simulink model "sampleModel3"  (R2023a)
settings: Solver=FixedStepAuto  StartTime=0.0  StopTime=10.0  RelTol=1e-3
undefined symbols (not defined in the file): DiscIntNeverNeededParam
libraries: simulink x8
settings Model: SimulationMode=software-in-the-loop (sil)  Creator=TSMC  LastModifiedBy=O
settings DataIOCC: InspectSignalLogs=on  SignalLoggingName=logsOut
settings OptimizationCC: DefaultParameterBehavior=Inlined  EnhancedBackFolding=on  PassReuseOutputArgsAs=Individual arguments  ZeroExternalMemoryAtStartup=off  ZeroInternalMemoryAtStartup=off  OptimizeBlockOrder=speed  DifferentSizesBufferReuse=on  OptimizationCustomize=off  EfficientTunableParamExpr=on
settings DebuggingCC: ParameterTunabilityLossMsg=error
settings ModelReferenceCC: UpdateModelReferenceTargets=Force
settings SFSimCC: MATLABDynamicMemAlloc=off
settings RTWCC: Description=Embedded Coder  SystemTargetFile=ert.tlc  TemplateMakefile=ert_default_tmf  GenerateReport=on  IncludeHyperlinkInReport=on  GenerateTraceInfo=on
settings CodeAppCC: ForceParamTrailComments=on  IgnoreCustomStorageClasses=off  OperatorAnnotations=on  SimulinkDataObjDesc=on  SFDataObjDesc=on  InsertBlockDesc=on
settings ERTTargetCC: TargetLangStandard=C99 (ISO)  GenerateSampleERTMain=on  SupportContinuousTime=on  InlinedParameterPlacement=NonHierarchical  ERTCustomFileTemplate=example_file_process.tlc

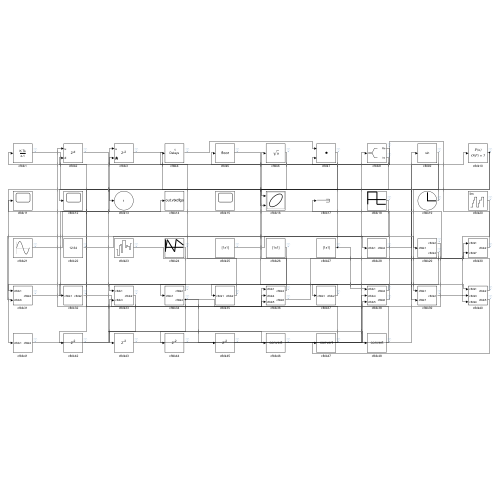
[thumbnail: Simulink's stored preview of the top-level diagram]
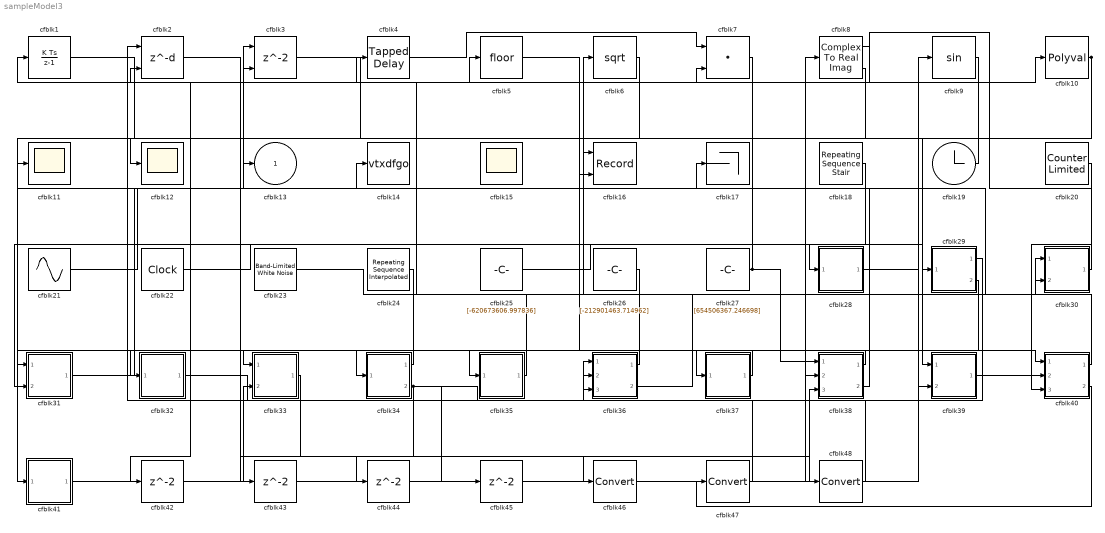
== system sampleModel3 ==
  cfblk1 : DiscreteIntegrator  ICPrevOutput=DiscIntNeverNeededParam  ICPrevScaledInput=DiscIntNeverNeededParam
  cfblk10 : Polyval  Coefs=[ +2.081618890e-019, -1.441693666e-014, +4.719686976e-010, -8.536869453e-006, +1.621573104e-001, -8.087801117e+001 ]
  cfblk11 : Scope
  cfblk12 : Scope
  cfblk14 : ToWorkspace  VariableName=vtxdfgo  SaveFormat=Timeseries  SampleTime=-1
  cfblk15 : Scope
      settings: Floating=on
  cfblk16 : Record  FileSettingsInternal="{\"entries\":[{\"content\":{\"excelSettings\":{\"content\":{},\"type\":\"Streamout.ExcelSettings\"}},\"type\":\"Streamout.FileSettingStorage\",\"uuid\":\"\"}],\"packageUris\":[\"http:\\/\\/schema.mathworks.com\\/mf0\\/streamout_blocks\\/R2020a\"],\"version\":\"1.0\"}"  Layout=[1 1]  SignalsInternal="{\"entries\":[{\"content\":{},\"type\":\"RecordBlkView.InputSignals\",\"uuid\":\"\"}],\"packageUris\":[\"http:\\/\\/schema.mathworks.com\\/mf0\\/streamout_blocks\\/R2020a\"],\"version\":\"1.0\"}"  VisualizationBindings="{\"xyplotplugin\":{\"info\":[{\"series\":[],\"subplotID\":1}]}}"  CompatibilityTag=XY
  cfblk17 : Terminator
  cfblk18 : simulink/Sources/Repeating Sequence Stair  OutValues=[683621746.226456, -425976951.351904]  tsamp=-1  OutMin=[]  OutMax=[]  OutDataTypeStr=double  OutputDataTypeScalingMode=double  OutDataType=fixdt(0,8)  ConRadixGroup=Best Precision: Vector-wise  OutScaling=2^-12
  cfblk19 : Clock
  cfblk2 : Delay  DelayLengthSource=Input port  SampleTime=1
      settings: InputPortMap=u0,p1
  cfblk20 : simulink/Sources/Counter Limited  uplimit=[952.000000]  tsamp=-1
  cfblk21 : Sin  Amplitude=[-7935361.579874]  Bias=[-620617910.021881]  SampleTime=0
  cfblk22 : DigitalClock
  cfblk23 : simulink/Sources/Band-Limited White Noise  Cov=[6099696625.296525]  Ts=0.1  seed=[892437433.000000]
  cfblk24 : simulink/Sources/Repeating Sequence Interpolated  OutValues=[-241246574.591498, 696589319.816223, -385466579.888859, 738540772.588338, 209128853.728495]  TimeValues=[0 0.1 0.5 0.6 1].'  LookUpMeth=Use Input Nearest  tsamp=0.01  OutMin=[]  OutMax=[]  OutDataTypeStr=double  OutputDataTypeScalingMode=double  OutDataType=fixdt(0,8)  OutScaling=2^-10
  cfblk25 : Constant  Value=[-620673606.997836]  SampleTime=1
  cfblk26 : Constant  Value=[-212901463.714962]  SampleTime=1
  cfblk27 : Constant  Value=[654506367.246698]  SampleTime=1
  cfblk28 : Subsystem
  cfblk29 : Subsystem
  cfblk3 : Delay  ShowEnablePort=on  SampleTime=1
      settings: InputPortMap=u0,e6
  cfblk30 : Subsystem
  cfblk31 : Subsystem
  cfblk32 : Subsystem
  cfblk33 : Subsystem
  cfblk34 : Subsystem
  cfblk35 : Subsystem
  cfblk36 : Subsystem
  cfblk37 : Subsystem
  cfblk38 : Subsystem
  cfblk39 : Subsystem
  cfblk4 : simulink/Discrete/Tapped Delay  vinit=0.0  samptime=-1  NumDelays=1  DelayOrder=Oldest  includeCurrent=off
  cfblk40 : Subsystem
  cfblk41 : Subsystem
  cfblk{42..45} (4 alike) : Delay  SampleTime=1
  cfblk46 : DataTypeConversion  SaturateOnIntegerOverflow=off  RndMeth=Floor
  cfblk47 : DataTypeConversion  SaturateOnIntegerOverflow=off  RndMeth=Floor
  cfblk48 : DataTypeConversion  SaturateOnIntegerOverflow=off  RndMeth=Floor
  cfblk5 : Rounding
  cfblk6 : Sqrt
  cfblk7 : DotProduct  OutDataTypeStr=Inherit: Inherit via internal rule
  cfblk8 : ComplexToRealImag
  cfblk9 : Trigonometry
  cfblk13 : Outport
  wires:
  cfblk31/1(cfblk2) -> cfblk14/1
  cfblk26/1 -> cfblk33/1(cfblk1)
  cfblk25/1 -> cfblk39/1(cfblk1)
  cfblk9/1 -> cfblk41/1(cfblk1)
  cfblk29/1(cfblk2) -> cfblk36/1(cfblk1)
  cfblk40/1(cfblk2) -> cfblk17/1
  cfblk22/1 -> cfblk28/1(cfblk1)
  cfblk29/2(cfblk4) -> cfblk35/1(cfblk1)
  cfblk3/1 -> cfblk39/2(cfblk7)
  cfblk30/1(cfblk2) -> cfblk5/1
  cfblk19/1 -> cfblk1/1
  cfblk35/1(cfblk2) -> cfblk4/1
  cfblk36/1(cfblk2) -> cfblk6/1
  cfblk21/1 -> cfblk3/1
  cfblk38/1(cfblk2) -> cfblk37/1(cfblk1)
  cfblk5/1 -> cfblk40/1(cfblk1)
  cfblk27/1 -> cfblk3/2, cfblk38/1(cfblk1)
  cfblk36/2(cfblk6) -> cfblk30/1(cfblk1)
  cfblk32/1(cfblk2) -> cfblk36/2(cfblk4)
  cfblk23/1 -> cfblk30/2(cfblk7)
  cfblk24/1 -> cfblk31/1(cfblk1)
  cfblk10/1 -> cfblk29/1(cfblk1), cfblk16/2
  cfblk4/1 -> cfblk7/1
  cfblk20/1 -> cfblk40/2(cfblk3)
  cfblk38/2(cfblk6) -> cfblk11/1
  cfblk41/1(cfblk2) -> cfblk33/2(cfblk3)
  cfblk1/1 -> cfblk13/1
  cfblk18/1 -> cfblk31/2(cfblk6)
  cfblk39/1(cfblk2) -> cfblk40/3(cfblk4)
  cfblk8/1 -> cfblk7/2
  cfblk7/1 -> cfblk16/1
  cfblk6/1 -> cfblk12/1
  cfblk28/1(cfblk2) -> cfblk10/1
  cfblk37/1(cfblk2) -> cfblk34/1(cfblk1)
  cfblk34/1(cfblk2) -> cfblk32/1(cfblk1)
  cfblk34/2(cfblk4) -> cfblk36/3(cfblk5), cfblk44/1, cfblk45/1
  cfblk8/2 -> cfblk42/1
  cfblk33/1(cfblk2) -> cfblk43/1
  cfblk43/1 -> cfblk9/1
  cfblk44/1 -> cfblk38/2(cfblk4)
  cfblk45/1 -> cfblk38/3(cfblk5)
  cfblk2/1 -> cfblk46/1
  cfblk46/1 -> cfblk8/1
  cfblk40/2(cfblk5) -> cfblk47/1
  cfblk47/1 -> cfblk2/1
  cfblk42/1 -> cfblk48/1
  cfblk48/1 -> cfblk2/2

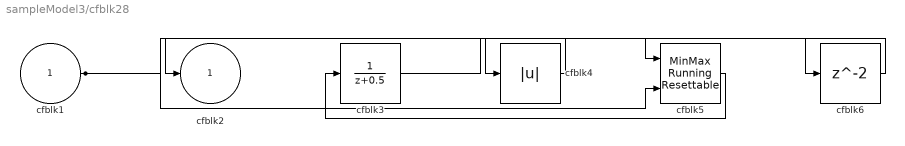
== system sampleModel3/cfblk28 ==
  cfblk1 : Inport
  cfblk3 : DiscreteTransferFcn  SampleTime=1
  cfblk4 : Abs  SaturateOnIntegerOverflow=off
  cfblk5 : simulink/Math Operations/MinMax Running Resettable  Function=min  vinit=0.0
  cfblk6 : Delay  SampleTime=1
  cfblk2 : Outport
  wires:
  cfblk4/1 -> cfblk2/1
  cfblk5/1 -> cfblk3/1
  cfblk1/1 -> cfblk5/2, cfblk4/1
  cfblk3/1 -> cfblk6/1
  cfblk6/1 -> cfblk5/1

== system sampleModel3/cfblk29 ==
  cfblk1 : Inport
  cfblk3 : Sum  Inputs=|++
  cfblk2 : Outport
  cfblk4 : Outport  Port=2
  wires:
  cfblk3/1 -> cfblk2/1
  cfblk1/1 -> cfblk4/1, cfblk3/1, cfblk3/2

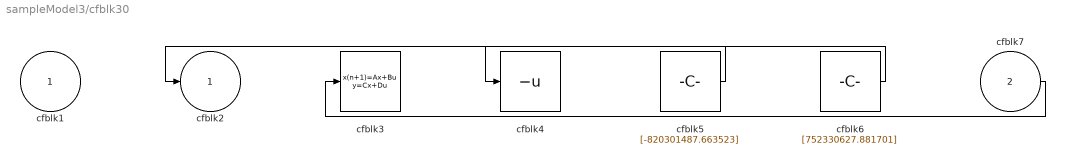
== system sampleModel3/cfblk30 ==
  cfblk1 : Inport
  cfblk7 : Inport  Port=2
  cfblk3 : DiscreteStateSpace
  cfblk4 : UnaryMinus
  cfblk5 : Constant  Value=[-820301487.663523]  SampleTime=1
  cfblk6 : Constant  Value=[752330627.881701]  SampleTime=1
  cfblk2 : Outport
  wires:
  cfblk6/1 -> cfblk4/1
  cfblk7/1 -> cfblk3/1
  cfblk5/1 -> cfblk2/1

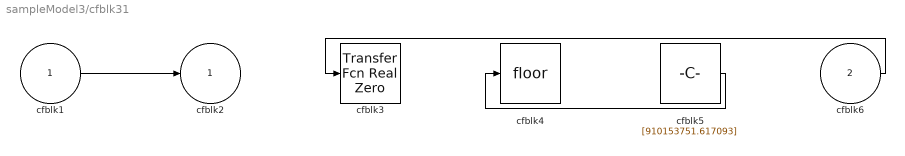
== system sampleModel3/cfblk31 ==
  cfblk1 : Inport
  cfblk6 : Inport  Port=2
  cfblk3 : simulink/Discrete/Transfer Fcn Real Zero  ZeroZ=0.75  ICPrevInput=0.0  DoSatur=off
  cfblk4 : Rounding
  cfblk5 : Constant  Value=[910153751.617093]  SampleTime=1
  cfblk2 : Outport
  wires:
  cfblk6/1 -> cfblk3/1
  cfblk5/1 -> cfblk4/1
  cfblk1/1 -> cfblk2/1

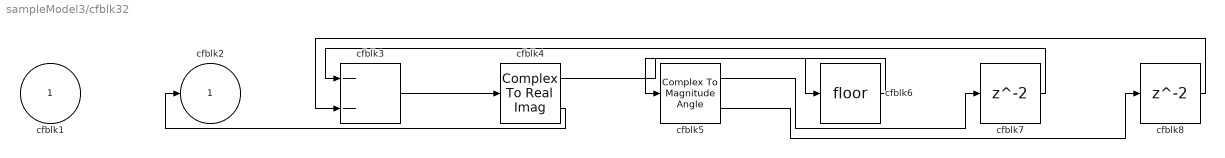
== system sampleModel3/cfblk32 ==
  cfblk1 : Inport
  cfblk3 : Sum  Inputs=--
  cfblk4 : ComplexToRealImag
  cfblk5 : ComplexToMagnitudeAngle
  cfblk6 : Rounding
  cfblk7 : Delay  SampleTime=1
  cfblk8 : Delay  SampleTime=1
  cfblk2 : Outport
  wires:
  cfblk6/1 -> cfblk5/1
  cfblk3/1 -> cfblk4/1
  cfblk4/1 -> cfblk6/1
  cfblk4/2 -> cfblk2/1
  cfblk5/1 -> cfblk7/1
  cfblk7/1 -> cfblk3/1
  cfblk5/2 -> cfblk8/1
  cfblk8/1 -> cfblk3/2

== system sampleModel3/cfblk33 ==
  cfblk1 : Inport
  cfblk3 : Inport  Port=2
  cfblk2 : Outport
  wires:
  cfblk1/1 -> cfblk2/1

== system sampleModel3/cfblk34 ==
  cfblk1 : Inport
  cfblk3 : Sum  Inputs=|++
  cfblk2 : Outport
  cfblk4 : Outport  Port=2
  wires:
  cfblk1/1 -> cfblk3/1, cfblk4/1, cfblk3/2
  cfblk3/1 -> cfblk2/1

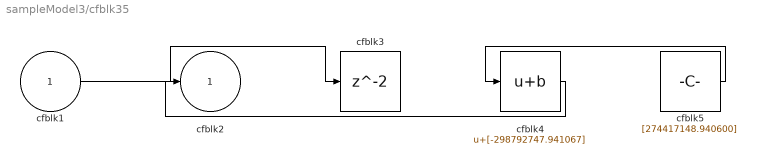
== system sampleModel3/cfblk35 ==
  cfblk1 : Inport
  cfblk3 : Delay  SampleTime=1
  cfblk4 : Bias  Bias=[-298792747.941067]  SaturateOnIntegerOverflow=off
  cfblk5 : Constant  Value=[274417148.940600]  SampleTime=1
  cfblk2 : Outport
  wires:
  cfblk5/1 -> cfblk4/1
  cfblk1/1 -> cfblk3/1
  cfblk4/1 -> cfblk2/1

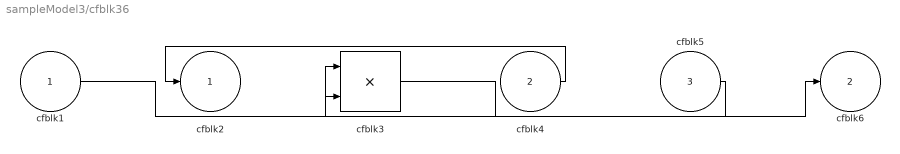
== system sampleModel3/cfblk36 ==
  cfblk1 : Inport
  cfblk4 : Inport  Port=2
  cfblk5 : Inport  Port=3
  cfblk3 : Product  Inputs=**
  cfblk2 : Outport
  cfblk6 : Outport  Port=2
  wires:
  cfblk4/1 -> cfblk2/1
  cfblk1/1 -> cfblk3/1
  cfblk3/1 -> cfblk6/1
  cfblk5/1 -> cfblk3/2

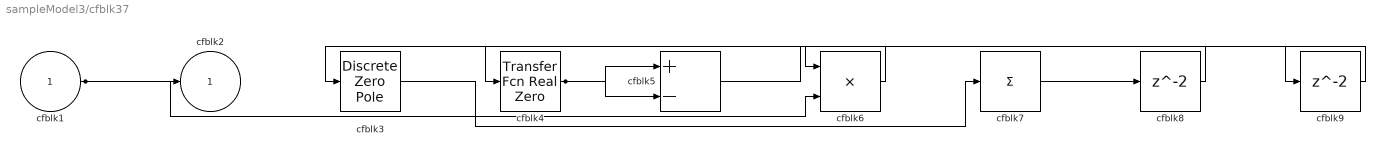
== system sampleModel3/cfblk37 ==
  cfblk1 : Inport
  cfblk3 : DiscreteZeroPole  Poles=[0 0.5]  Gain=1
  cfblk4 : simulink/Discrete/Transfer Fcn Real Zero  ZeroZ=0.75  ICPrevInput=0.0  DoSatur=off
  cfblk5 : Sum  Inputs=+-
  cfblk6 : Product
  cfblk7 : Sum  Inputs=+
  cfblk8 : Delay  SampleTime=1
  cfblk9 : Delay  SampleTime=1
  cfblk2 : Outport
  wires:
  cfblk6/1 -> cfblk3/1
  cfblk3/1 -> cfblk7/1
  cfblk4/1 -> cfblk5/1, cfblk5/2
  cfblk1/1 -> cfblk6/2, cfblk2/1
  cfblk7/1 -> cfblk8/1
  cfblk8/1 -> cfblk6/1
  cfblk5/1 -> cfblk9/1
  cfblk9/1 -> cfblk4/1

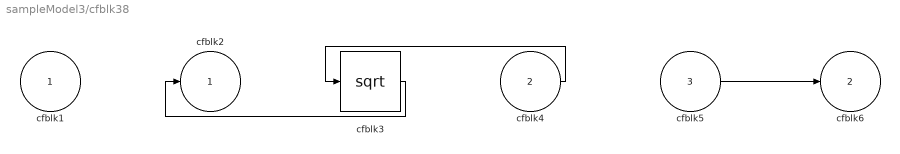
== system sampleModel3/cfblk38 ==
  cfblk1 : Inport
  cfblk4 : Inport  Port=2
  cfblk5 : Inport  Port=3
  cfblk3 : Sqrt
  cfblk2 : Outport
  cfblk6 : Outport  Port=2
  wires:
  cfblk5/1 -> cfblk6/1
  cfblk4/1 -> cfblk3/1
  cfblk3/1 -> cfblk2/1

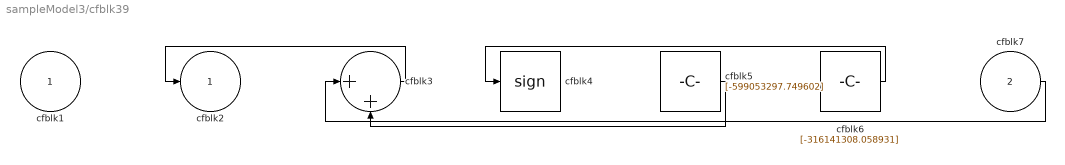
== system sampleModel3/cfblk39 ==
  cfblk1 : Inport
  cfblk7 : Inport  Port=2
  cfblk3 : Sum  Inputs=|++
  cfblk4 : Signum
  cfblk5 : Constant  Value=[-599053297.749602]  SampleTime=1
  cfblk6 : Constant  Value=[-316141308.058931]  SampleTime=1
  cfblk2 : Outport
  wires:
  cfblk6/1 -> cfblk4/1
  cfblk7/1 -> cfblk3/1
  cfblk5/1 -> cfblk3/2
  cfblk3/1 -> cfblk2/1

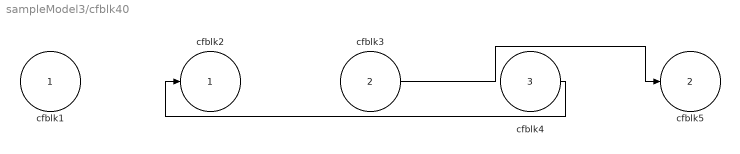
== system sampleModel3/cfblk40 ==
  cfblk1 : Inport
  cfblk3 : Inport  Port=2
  cfblk4 : Inport  Port=3
  cfblk2 : Outport
  cfblk5 : Outport  Port=2
  wires:
  cfblk3/1 -> cfblk5/1
  cfblk4/1 -> cfblk2/1

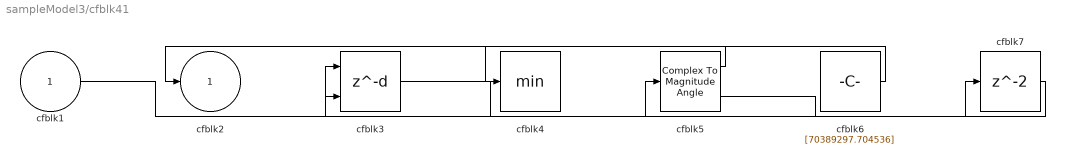
== system sampleModel3/cfblk41 ==
  cfblk1 : Inport
  cfblk3 : Delay  DelayLengthSource=Input port  SampleTime=1
      settings: InputPortMap=u0,p1
  cfblk4 : MinMax
  cfblk5 : ComplexToMagnitudeAngle
  cfblk6 : Constant  Value=[70389297.704536]  SampleTime=1
  cfblk7 : Delay  SampleTime=1
  cfblk2 : Outport
  wires:
  cfblk5/1 -> cfblk2/1
  cfblk1/1 -> cfblk3/1
  cfblk3/1 -> cfblk5/1
  cfblk6/1 -> cfblk4/1
  cfblk5/2 -> cfblk7/1
  cfblk7/1 -> cfblk3/2
